simulink library "DSMLib"  (R2016b)
settings: Solver=VariableStepAuto  StartTime=0.0  StopTime=10.0  RelTol=1e-3
settings Model: Creator=Administrator  LastModifiedBy=muou

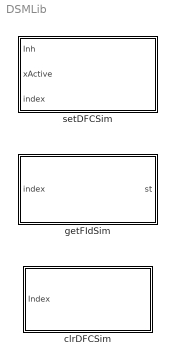
== system DSMLib ==
  clrDFCSim : Subsystem
  getFIdSim : Subsystem
  setDFCSim : Subsystem

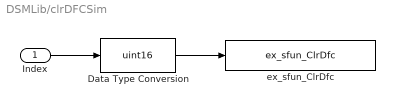
== system DSMLib/clrDFCSim ==
  Index : Inport
  Data Type Conversion : DataTypeConversion  OutDataTypeStr=uint16
  ex_sfun_ClrDfc : S-Function  FunctionName=ex_sfun_ClrDfc  SFunctionDeploymentMode=off  EnableBusSupport=off  mask(Legacy Function){SFunctionSpec=void ClrDfcShell(uint16 u1), ShowSpec=on}
      mask prompts: ShowSpec "Display function specification"
      mask help:
      | This block allows you to call the legacy functions specified by the following Legacy Code Tool definition:
      | def.SFunctionName = 'ex_sfun_ClrDfc';
      | def.OutputFcnSpec = 'void ClrDfcShell(uint16 u1)';
      | def.HeaderFiles = {'C2SfunShell.h', 'Platform_Types.h', 'LIB_Atan2.h', 'LIB_SinCosCalc.h', 'LIB_SqrtCalc.h'};
      | def.SourceFiles = {'C2SfunShell.c', 'LIB_Atan2.c', 'LIB_SinCosCalc.c', 'LIB_SqrtCalc.c'};
      mask Help: <p>This block was generated automatically by the Legacy Code Tool. For detailed help on this tool, call<a href="matlab:legacy_code('help')"> legacy_code('help')</a>.</p>
      mask Callback ShowSpec:
      | if strcmp(get_param(gcbh, 'ShowSpec'), 'on')
      |   set_param(gcbh, 'MaskDisplay', sprintf('fprintf(''%s'');', get_param(gcbh, 'SFunctionSpec')));
      | else
      |   set_param(gcbh, 'MaskDisplay', sprintf('fprintf(''%s'');', get_param(gcbh, 'FunctionName')));
      | end
      mask Display: fprintf('%s','void ClrDfcShell(uint16 u1)');
  wires:
  Data Type Conversion/1 -> ex_sfun_ClrDfc/1
  Index/1 -> Data Type Conversion/1

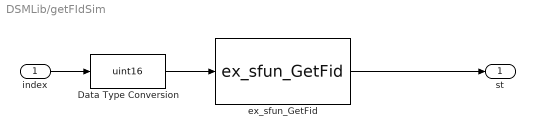
== system DSMLib/getFIdSim ==
  index : Inport
  Data Type Conversion : DataTypeConversion  OutDataTypeStr=uint16
  ex_sfun_GetFid : S-Function  FunctionName=ex_sfun_GetFid  SFunctionDeploymentMode=off  EnableBusSupport=off  mask(Legacy Function){SFunctionSpec=void GetFidShell(uint16 u1,boolean y1[1]), ShowSpec=on}
      mask prompts: ShowSpec "Display function specification"
      mask help:
      | This block allows you to call the legacy functions specified by the following Legacy Code Tool definition:
      | def.SFunctionName = 'ex_sfun_GetFid';
      | def.OutputFcnSpec = 'void GetFidShell(uint16 u1,boolean y1[1])';
      | def.HeaderFiles = {'C2SfunShell.h', 'Platform_Types.h', 'LIB_Atan2.h', 'LIB_SinCosCalc.h', 'LIB_SqrtCalc.h'};
      | def.SourceFiles = {'C2SfunShell.c', 'LIB_Atan2.c', 'LIB_SinCosCalc.c', 'LIB_SqrtCalc.c'};
      mask Help: <p>This block was generated automatically by the Legacy Code Tool. For detailed help on this tool, call<a href="matlab:legacy_code('help')"> legacy_code('help')</a>.</p>
      mask Callback ShowSpec:
      | if strcmp(get_param(gcbh, 'ShowSpec'), 'on')
      |   set_param(gcbh, 'MaskDisplay', sprintf('fprintf(''%s'');', get_param(gcbh, 'SFunctionSpec')));
      | else
      |   set_param(gcbh, 'MaskDisplay', sprintf('fprintf(''%s'');', get_param(gcbh, 'FunctionName')));
      | end
      mask Display: fprintf('GetFidShell\n (uint16 u1,boolean y1[1])');
  st : Outport
  wires:
  index/1 -> Data Type Conversion/1
  ex_sfun_GetFid/1 -> st/1
  Data Type Conversion/1 -> ex_sfun_GetFid/1

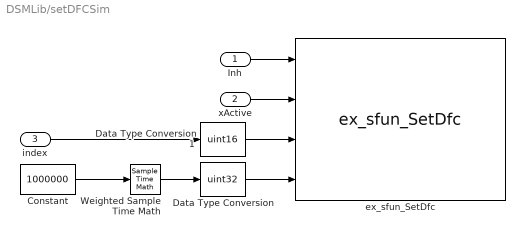
== system DSMLib/setDFCSim ==
  Inh : Inport
  xActive : Inport  Port=2
  index : Inport  Port=3
  Constant : Constant  Value=1000000
  Data Type Conversion : DataTypeConversion  OutDataTypeStr=uint32
  Data Type Conversion1 : DataTypeConversion  OutDataTypeStr=uint16
  Weighted Sample Time Math : SampleTimeMath  TsampMathOp=*  TsampMathImp=Offline Scaling Adjustment
  ex_sfun_SetDfc : S-Function  FunctionName=ex_sfun_SetDfc  SFunctionDeploymentMode=off  EnableBusSupport=off  mask(Legacy Function){SFunctionSpec=void SetDfcShell(boolean u1,boolean u2, uint16 u3, uint32 u4), ShowSpec=on}
      mask prompts: ShowSpec "Display function specification"
      mask help:
      | This block allows you to call the legacy functions specified by the following Legacy Code Tool definition:
      | def.SFunctionName = 'ex_sfun_SetDfc';
      | def.OutputFcnSpec = 'void SetDfcShell(boolean u1,boolean u2, uint16 u3, uint32 u4)';
      | def.HeaderFiles = {'C2SfunShell.h', 'Platform_Types.h', 'LIB_Atan2.h', 'LIB_SinCosCalc.h', 'LIB_SqrtCalc.h'};
      | def.SourceFiles = {'C2SfunShell.c', 'LIB_Atan2.c', 'LIB_SinCosCalc.c', 'LIB_SqrtCalc.c'};
      mask Help: <p>This block was generated automatically by the Legacy Code Tool. For detailed help on this tool, call<a href="matlab:legacy_code('help')"> legacy_code('help')</a>.</p>
      mask Callback ShowSpec:
      | if strcmp(get_param(gcbh, 'ShowSpec'), 'on')
      |   set_param(gcbh, 'MaskDisplay', sprintf('fprintf(''%s'');', get_param(gcbh, 'SFunctionSpec')));
      | else
      |   set_param(gcbh, 'MaskDisplay', sprintf('fprintf(''%s'');', get_param(gcbh, 'FunctionName')));
      | end
      mask Display: fprintf('%s',' SetDfcShell\nInh,xActive, Idx, debouceTime');
  wires:
  Constant/1 -> Weighted Sample Time Math/1
  Data Type Conversion/1 -> ex_sfun_SetDfc/4
  Weighted Sample Time Math/1 -> Data Type Conversion/1
  Inh/1 -> ex_sfun_SetDfc/1
  xActive/1 -> ex_sfun_SetDfc/2
  index/1 -> Data Type Conversion1/1
  Data Type Conversion1/1 -> ex_sfun_SetDfc/3
